simulink subsystem "SerializeINT16"  (R2019b)
settings: Solver=VariableStepAuto  StartTime=0.0  StopTime=10.0  RelTol=1e-3
settings Model: Creator=VM  LastModifiedBy=VM

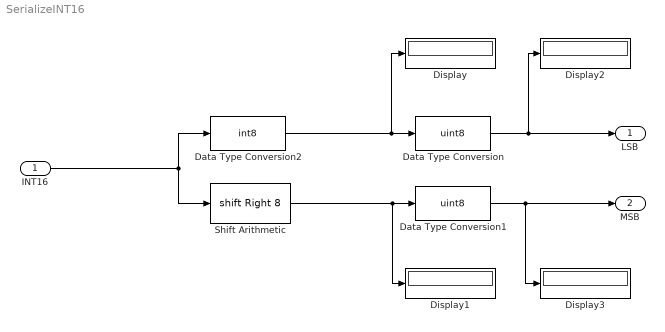
== system SerializeINT16 ==
  INT16 : Inport  OutDataTypeStr=int16
  Data Type Conversion : DataTypeConversion  OutDataTypeStr=uint8
  Data Type Conversion1 : DataTypeConversion  OutDataTypeStr=uint8
  Data Type Conversion2 : DataTypeConversion  OutDataTypeStr=int8  ConvertRealWorld=Stored Integer (SI)
  Display{,1..3} (4 alike) : Display
  Shift Arithmetic : ArithShift  BitShiftNumber=8  BitShiftDirection=Right
  LSB : Outport
  MSB : Outport  Port=2
  wires:
  Data Type Conversion2/1 -> Data Type Conversion/1, Display/1
  INT16/1 -> Shift Arithmetic/1, Data Type Conversion2/1
  Shift Arithmetic/1 -> Data Type Conversion1/1, Display1/1
  Data Type Conversion1/1 -> MSB/1, Display3/1
  Data Type Conversion/1 -> LSB/1, Display2/1
